simulink model "Sector_Caculate"  (R2024b)
settings: Solver=VariableStepAuto  StartTime=0.0  StopTime=10.0  RelTol=1e-3
settings Model: Creator=罗芳成  LastModifiedBy=罗芳成

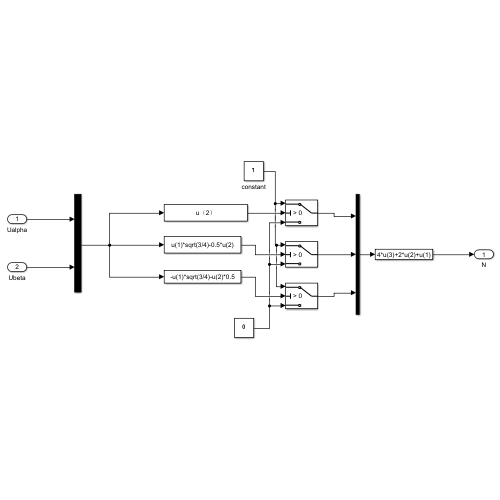
[thumbnail: Simulink's stored preview of the top-level diagram]
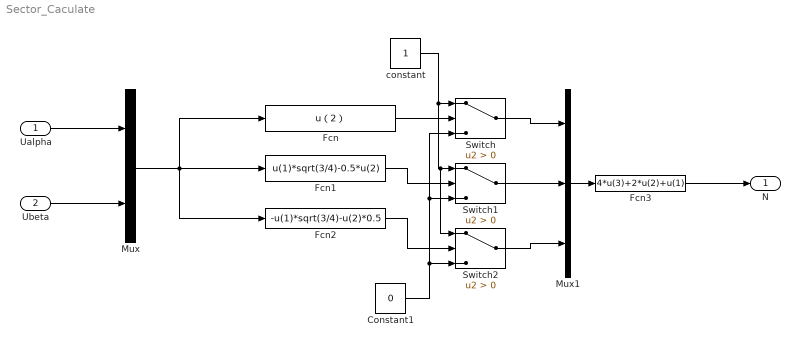
== system Sector_Caculate ==
  Ualpha : Inport
  Ubeta : Inport  Port=2
  Constant1 : Constant  Value=0
  Fcn : Fcn  Expr=u（2）
  Fcn1 : Fcn  Expr=u(1)*sqrt(3/4)-0.5*u(2)
  Fcn2 : Fcn  Expr=-u(1)*sqrt(3/4)-u(2)*0.5
  Fcn3 : Fcn  Expr=4*u(3)+2*u(2)+u(1)
  Mux : Mux  Inputs=2
  Mux1 : Mux  Inputs=3
  Switch : Switch  Criteria=u2 > Threshold  SaturateOnIntegerOverflow=off  InputSameDT=off
  Switch1 : Switch  Criteria=u2 > Threshold  SaturateOnIntegerOverflow=off  InputSameDT=off
  Switch2 : Switch  Criteria=u2 > Threshold  SaturateOnIntegerOverflow=off  InputSameDT=off
  constant : Constant
  N : Outport
  wires:
  Switch2/1 -> Mux1/3
  Fcn/1 -> Switch/2
  Fcn2/1 -> Switch2/2
  Ubeta/1 -> Mux/2
  Switch1/1 -> Mux1/2
  Switch/1 -> Mux1/1
  Fcn1/1 -> Switch1/2
  Constant1/1 -> Switch/3, Switch1/3, Switch2/3
  constant/1 -> Switch2/1, Switch1/1, Switch/1
  Mux/1 -> Fcn/1, Fcn2/1, Fcn1/1
  Ualpha/1 -> Mux/1
  Mux1/1 -> Fcn3/1
  Fcn3/1 -> N/1
